simulink model "Gyroscope_Model"  (R2020b)
settings: Solver=VariableStepAuto  StartTime=0.0  StopTime=50  RelTol=1e-3
values from neighbouring files (symbols this model uses):
  A = [0 1 0 0 0 0 ... (first row only)    [Gyro.m]    (also in VortexNoise.m = A/0.3048^2)
  B = [0 0 0 0 0 0 ... (first row only)    [Gyro.m]
  C = eye(6)    [Gyro.m]
  D = zeros(6)    [Gyro.m]
  phi_0 = 0    [Gyro.m]
  phi_d_0 = 0.1    [Gyro.m]
  psi_0 = 0    [Gyro.m]
  psi_d_0 = 0    [Gyro.m]
  theta_0 = 20*pi/180    (= 0.349065850399)    [Gyro.m]    (also in Propellers_tilt.m = [0; 0; 0]; six.m = [0;0;0]; tilt_verification.m = [0; 0; 0])
  theta_d_0 = 0.1    [Gyro.m]
libraries: pid_lib x1
settings Model: Creator=Jonathan van Zyl  LastModifiedBy=Jonathan van Zyl

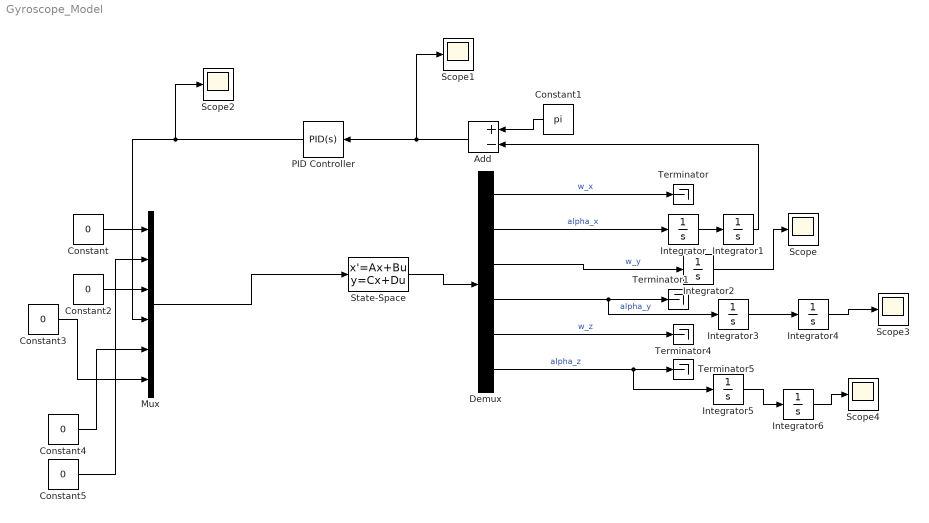
== system Gyroscope_Model ==
  Add : Sum  Inputs=+-
  Constant{,2..5} (5 alike) : Constant  Value=0
  Constant1 : Constant  Value=pi
  Demux : Demux  Outputs=6
  Integrator : Integrator  InitialCondition=theta_d_0
  Integrator1 : Integrator  InitialCondition=theta_0
  Integrator2 : Integrator
  Integrator3 : Integrator  InitialCondition=phi_d_0
  Integrator4 : Integrator  InitialCondition=phi_0
  Integrator5 : Integrator  InitialCondition=psi_d_0
  Integrator6 : Integrator  InitialCondition=psi_0
  Mux : Mux  Inputs=6
  PID Controller : pid_lib/PID Controller  Controller=PID  Form=Parallel  TimeDomain=Continuous-time  UseExternalTs=off  SampleTime=-1  IntegratorMethod=Forward Euler  FilterMethod=Forward Euler  ControllerParametersSource=internal  P=0.296738839189935  I=0.0106852580966872  D=1.20174097843501  UseFilter=on  N=11.3634813848559  TunerSelectOption=Transfer Function Based (PID Tuner App)  InitialConditionSource=internal  InitialConditionForIntegrator=0  InitialConditionForFilter=0  DifferentiatorICPrevScaledInput=0  ExternalReset=none  TrackingMode=off  Kt=1  LimitOutput=off  SatLimitsSource=internal  UpperSaturationLimit=inf  LowerSaturationLimit=-inf  LinearizeAsGain=on  AntiWindupMode=none  Kb=1  POutMin=[]  POutMax=[]  IOutMin=[]  IOutMax=[]  DOutMin=[]  DOutMax=[]  NOutMin=[]  NOutMax=[]  SumOutMin=[]  SumOutMax=[]  SaturationOutMin=[]  SaturationOutMax=[]  PParamMin=[]  PParamMax=[]  IParamMin=[]  IParamMax=[]  DParamMin=[]  DParamMax=[]  NParamMin=[]  NParamMax=[]  KbParamMin=[]  KbParamMax=[]  KtParamMin=[]  KtParamMax=[]  KbOutMin=[]  KbOutMax=[]  KtOutMin=[]  KtOutMax=[]  IntegratorOutMin=[]  IntegratorOutMax=[]  FilterOutMin=[]  FilterOutMax=[]  SumI1OutMin=[]  SumI1OutMax=[]  SumI2OutMin=[]  SumI2OutMax=[]  SumI3OutMin=[]  SumI3OutMax=[]  SumI4OutMin=[]  SumI4OutMax=[]  SumDOutMin=[]  SumDOutMax=[]  DifferentiatorOutMin=[]  DifferentiatorOutMax=[]  FilterDiffOutCoefMin=[]  FilterDiffOutCoefMax=[]  ReciprocalOutMin=[]  ReciprocalOutMax=[]  SumDenOutMin=[]  SumDenOutMax=[]  SumNumOutMin=[]  SumNumOutMax=[]  DivideOutMin=[]  DivideOutMax=[]  UdiffTsProdOutMin=[]  UdiffTsProdOutMax=[]  NTsProdOutMin=[]  NTsProdOutMax=[]  UintegralTsProdOutMin=[]  UintegralTsProdOutMax=[]  UngainTsProdOutMin=[]  UngainTsProdOutMax=[]  IntegratorContinuousStateAttributes=''  IntegratorStateMustResolveToSignalObject=off  IntegratorRTWStateStorageClass=Auto  FilterContinuousStateAttributes=''  FilterStateMustResolveToSignalObject=off  FilterRTWStateStorageClass=Auto  ParallelPVariant=InternalParameters  IdealPVariant=Disabled  IVariant=InternalParameters  DVariant=InternalParameters  IntegratorVariant=Continuous  SatVariant=Disabled  AWVariant=Passthrough  PCopyVariant=Disabled  TRVariant=Disabled  FdbkBlocksVariant=Forward  IdealPFdbkVariant=Disabled  SatFdbkVariant=Disabled  DerivativeFilterVariant=ContFilter  NVariant=InternalParameters  NCopyVariant=Disabled  FilterICVariant=InternalICsFilter  IntegratorICVariant=InternalICs  ExternalResetVariant=Disabled  TRSumVariant=Passthrough  SumFdbkVariant=Disabled  SumVariant=Sum_PID  TsampFilterVariant=InternalTs  TsampNgainVariant=Passthrough  TsampIntegralVariant=Passthrough  ExternalSaturationOutDataTypeStr=Inherit: Same as second input
  Scope{,1..4} (5 alike) : Scope
  State-Space : StateSpace  A=A  B=B  C=C  D=D  InitialCondition=0
  Terminator{,1,4..5} (4 alike) : Terminator
  wires:
  Constant/1 -> Mux/1
  Constant2/1 -> Mux/3
  Constant4/1 -> Mux/5
  Mux/1 -> State-Space/1
  State-Space/1 -> Demux/1
  Demux/1 -> Terminator/1  "w_x"
  Demux/2 -> Integrator/1  "alpha_x"
  Demux/3 -> Integrator2/1  "w_y"
  Demux/4 -> Integrator3/1, Terminator1/1  "alpha_y"
  Demux/5 -> Terminator4/1  "w_z"
  Demux/6 -> Integrator5/1, Terminator5/1  "alpha_z"
  Integrator/1 -> Integrator1/1
  Constant1/1 -> Add/1
  Add/1 -> Scope1/1, PID Controller/1
  Constant3/1 -> Mux/6
  PID Controller/1 -> Mux/4, Scope2/1
  Integrator1/1 -> Add/2
  Integrator2/1 -> Scope/1
  Integrator3/1 -> Integrator4/1
  Integrator4/1 -> Scope3/1
  Integrator5/1 -> Integrator6/1
  Integrator6/1 -> Scope4/1
  Constant5/1 -> Mux/2
